simulink library "p1lib"  (R2018b)
settings: Solver=VariableStepAuto  StartTime=0.0  StopTime=10.0  RelTol=1e-3  EnableMultiTasking=on
values from neighbouring files (symbols this model uses):
  C_0 = 0.015    [init.m]
  C_D = 0.35    [init.m]
  eta_ess = 0.7    [init.m]
  g = 9.8    [init.m]
  G_diff = 0.25    [init.m]
  g_hr_to_gal_s = 9.778e-8    (= 9.778e-08)    [init.m]
  m_to_mi = 1/1609    (= 0.000621504039776)    [init.m]
  M_veh = 1746    [init.m]
  mph_to_mps = 0.44704    [init.m]
  r_wheel = 0.2794    [init.m]
  rho = 1.225    [init.m]
  SOC_init = 0.5    [init.m]
undefined symbols (not defined in the file or in its folder): E_max, eng_map, us06
settings Model: Creator=wasynczu  LastModifiedBy=wasynczu
settings DataIOCC: LimitDataPoints=on
settings OptimizationCC: LifeSpan=inf
settings DebuggingCC: AllowSymbolicDim=off  SFUnexpectedBacktrackingDiag=warning  SFNoUnconditionalDefaultTransitionDiag=warning  SFExecutionAtInitializationDiag=none
settings ModelReferenceCC: PropagateSignalLabelsOutOfModel=off
settings SFSimCC: SimUseLocalCustomCode=off
settings RTWCC: RTWUseLocalCustomCode=off
settings CodeAppCC: StateflowObjectComments=on
settings GRTTargetCC: TargetLangStandard=C89/C90 (ANSI)
settings ConfigComp: CovMetricSettings=dw  CovHtmlReporting=on  CovSaveCumulativeToWorkspaceVar=on  CovSaveSingleToWorkspaceVar=on  CovExternalEMLEnable=off

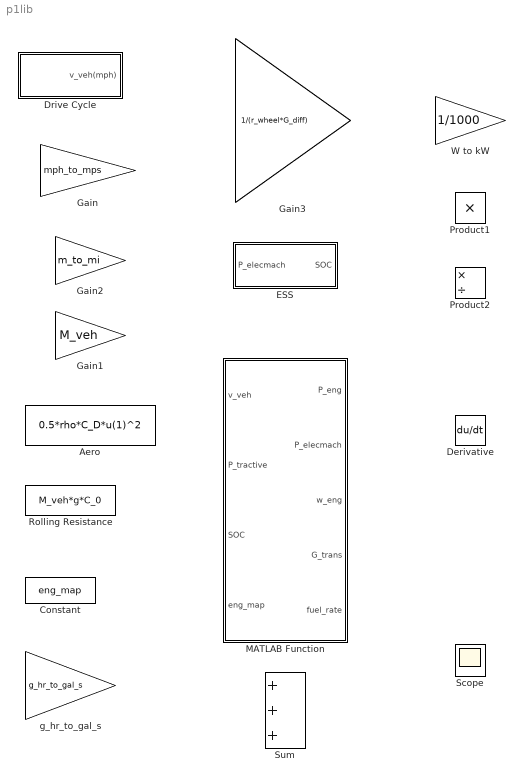
== system p1lib ==
  Aero : Fcn  Expr=0.5*rho*C_D*u(1)^2
  Constant : Constant  Value=eng_map
  Derivative : Derivative
  Drive Cycle : Subsystem  mask{schedule=us06}
      mask prompts: schedule "drive schedule"
      mask init:
      | N=length(schedule(:,1))
  ESS : Subsystem  mask{E_max=E_max, eta_ess=eta_ess}
      mask prompts: E_max "Maximum energy, J"; eta_ess "round-trip efficiency"
  Gain : Gain  Gain=mph_to_mps
  Gain1 : Gain  Gain=M_veh
  Gain2 : Gain  Gain=m_to_mi
  Gain3 : Gain  Gain=1/(r_wheel*G_diff)
  MATLAB Function : MATLAB Function  TreatAsAtomicUnit=on
  Product1 : Product
  Product2 : Product  Inputs=*/
  Rolling Resistance : Constant  Value=M_veh*g*C_0
  Scope : Scope
  Sum : Sum  Inputs=+++
  W to kW : Gain  Gain=1/1000
  g_hr_to_gal_s : Gain  Gain=g_hr_to_gal_s

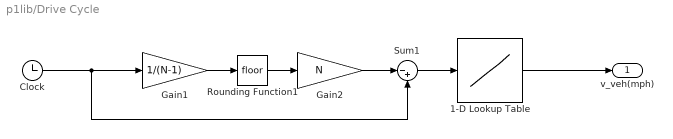
== system p1lib/Drive Cycle ==
  1-D Lookup Table : Lookup_n-D  NumberOfTableDimensions=1  BreakpointsForDimension1=schedule(:,1)  Table=schedule(:,2)  InternalRulePriority=Speed  RndMeth=Simplest  InputSameDT=on
  Clock : Clock
  Gain1 : Gain  Gain=1/(N-1)
  Gain2 : Gain  Gain=N
  Rounding Function1 : Rounding
  Sum1 : Sum  Inputs=|-+
  v_veh(mph) : Outport
  wires:
  Gain1/1 -> Rounding Function1/1
  Rounding Function1/1 -> Gain2/1
  Gain2/1 -> Sum1/1
  Sum1/1 -> 1-D Lookup Table/1
  Clock/1 -> Sum1/2, Gain1/1
  1-D Lookup Table/1 -> v_veh(mph)/1

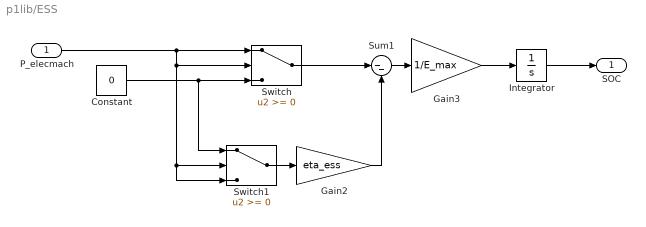
== system p1lib/ESS ==
  P_elecmach : Inport
  Constant : Constant  Value=0
  Gain2 : Gain  Gain=eta_ess
  Gain3 : Gain  Gain=1/E_max  OutDataTypeStr=fixdt('double', 'DataTypeOverride', 'Off')
  Integrator : Integrator  InitialCondition=SOC_init  LimitOutput=on  UpperSaturationLimit=1  LowerSaturationLimit=0
  Sum1 : Sum  Inputs=|--
  Switch : Switch  OutDataTypeStr=double
  Switch1 : Switch  OutDataTypeStr=double
  SOC : Outport
  wires:
  Integrator/1 -> SOC/1
  Constant/1 -> Switch/3, Switch1/1
  Switch/1 -> Sum1/1
  Sum1/1 -> Gain3/1
  Switch1/1 -> Gain2/1
  Gain2/1 -> Sum1/2
  Gain3/1 -> Integrator/1
  P_elecmach/1 -> Switch/1, Switch/2, Switch1/3, Switch1/2

== matlab function p1lib/MATLAB Function ==
  data: v_veh input; P_eng output; P_tractive input; SOC input; P_elecmach output; w_eng output; eng_map input; G_trans output; fuel_rate output
function [P_eng, P_elecmach, w_eng, G_trans, fuel_rate] = fcn(v_veh, P_tractive, SOC, eng_map)
%#codegen

v_min = 2.19;  % minimum vehicle speed for engine to stay engaged, in m/s
P_min = 10000; % minimum engine power in W
P_max = 80000; % maximum engine power
G_trans_min = 0.3; % minimum transmission gear ratio
G_diff = 0.25;    % differential gear ratio
r_wheel = 0.2794; % wheel radius in m


bsfc = 0;
if (v_veh < v_min)  % low-speed acceleration
   P_elecmach = P_tractive;
   P_eng = 0;
   fuel_rate = 0;
   w_eng = 0;
   G_trans = G_trans_min;
   return  
   
end

if(P_tractive < P_min)   % low-tractive-power, turn engine off
   P_elecmach = P_tractive;
   fuel_rate = 0;
   w_eng = 0;
   P_eng = 0;
   G_trans = G_trans_min;
   return     
end


if(P_tractive > P_max) %high-speed boost
   P_elecmach = P_tractive-P_max;
   P_eng = P_max;
   bsfc = interp1(eng_map(:,2), eng_map(:,3), P_eng/1000);
   fuel_rate = bsfc*P_eng/1000; % g/hr
   w_eng = interp1(eng_map(:,2), eng_map(:,1), P_eng/1000);
   w_rad_p_s = w_eng*pi/30; % convert to rad/s
   G_trans =  v_veh/r_wheel/G_diff/w_rad_p_s;
   return   
end
% charge sustaining mode
P_elecmach = -(P_max-P_tractive)*(0.5-SOC);
P_eng = P_tractive-P_elecmach;
bsfc = interp1(eng_map(:,2), eng_map(:,3), P_eng/1000);
fuel_rate = bsfc*P_eng/1000; % g/hr

w_eng = interp1(eng_map(:,2), eng_map(:,1), P_eng/1000);
w_rad_p_s = w_eng*pi/30;  % convert to rad/s
G_trans =  v_veh/r_wheel/G_diff/w_rad_p_s;

if(P_eng<P_min) % sshut it off
   P_eng = 0;
   P_elecmach = P_tractive;
   fuel_rate = 0;
   w_eng = 0;
   G_trans = G_trans_min;
   return
end
